simulink model "ELECTRONICSPEEDCONTROLLER"  (R2022b)
settings: Solver=VariableStepAuto  StartTime=0.0  StopTime=10.0  RelTol=1e-3
settings Model: Creator=lucaerviati  LastModifiedBy=lucaerviati
settings DataIOCC: SaveOutput=off  SaveTime=off
settings GRTTargetCC: CombineOutputUpdateFcns=off  MatFileLogging=off

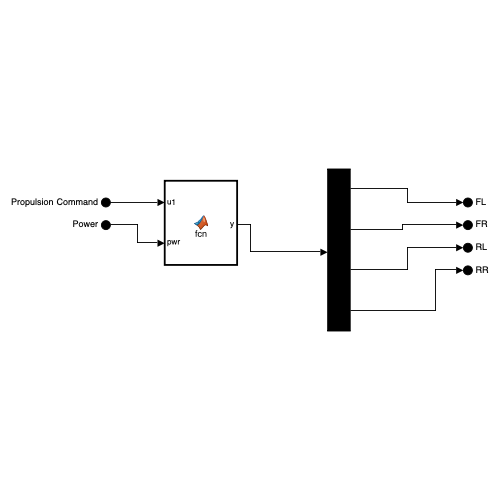
[thumbnail: Simulink's stored preview of the top-level diagram]
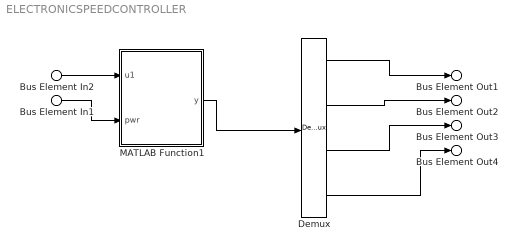
== system ELECTRONICSPEEDCONTROLLER ==
  Bus Element In2 : Inport  PortName=Propulsion Command
  Bus Element In1 : Inport  Port=2  PortName=Power
  Demux : Demux
  MATLAB Function1 : MATLAB Function  TreatAsAtomicUnit=on
  Bus Element Out1 : Outport  PortName=FL
  Bus Element Out2 : Outport  Port=2  PortName=FR
  Bus Element Out3 : Outport  Port=3  PortName=RL
  Bus Element Out4 : Outport  Port=4  PortName=RR
  wires:
  Demux/1 -> Bus Element Out1/1
  Demux/2 -> Bus Element Out2/1
  Demux/3 -> Bus Element Out3/1
  Demux/4 -> Bus Element Out4/1
  MATLAB Function1/1(y) -> Demux/1
  Bus Element In2/1 -> MATLAB Function1/1(u1)
  Bus Element In1/1 -> MATLAB Function1/2(pwr)

== matlab function ELECTRONICSPEEDCONTROLLER/MATLAB Function1 ==
  data: u1 input; y output; pwr input
function y = fcn(u1, pwr)

u = u1;


y = u*pwr;
